simulink model "SemiActive_TS9"  (Simulink 7.6)
settings: Solver=ode45  SolverMode=SingleTasking  StartTime=0  StopTime=20  FixedStep=0.001  RelTol=1e-3  AbsTol=1e-6
libraries: Solver_SF x1
settings Model: Creator=bduprey  LastModifiedBy=mkhan  ExtModeTrigMode=oneshot  ExtModeArmWhenConnect=off
settings DataIOCC: LimitDataPoints=off  SignalLoggingName=sigsOut
settings OptimizationCC: BooleanDataType=off
settings DebuggingCC: SaveWithParameterizedLinksMsg=none  SignalResolutionControl=TryResolveAllWithWarning  SolverPrmCheckMsg=none  MultiTaskDSMMsg=warning  MultiTaskCondExecSysMsg=none  StrictBusMsg=None
settings HardwareCC: TargetUnknown=on
settings RTWCC: TemplateMakefile=grt_vc.tmf  IncludeERTFirstTime=on

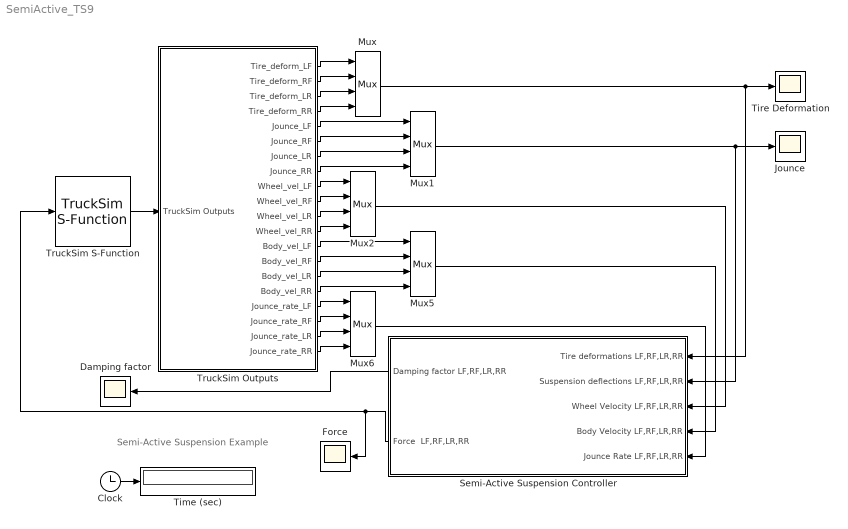
== system SemiActive_TS9 ==
  note: Semi-Active Suspension Example
  Clock : Clock
      settings: Decimation=10
  Damping factor : Scope
      settings: TickLabels=on  YMin=0  YMax=80000  DataFormat=Array  SampleTime=100
  Force : Scope
      settings: TickLabels=on  YMin=-100000  YMax=100000  DataFormat=Array  SampleTime=100
  Jounce : Scope
      settings: TickLabels=on  YMin=-0.1  YMax=0.3  DataFormat=Array  SampleTime=100
  Mux{,1..2,5..6} (5 alike) : Mux
  Semi-Active Suspension Controller : Subsystem  mask{K1=884.4, K1_R=679.6, K2=8624.1, K2_R=8624.1, K3=1398.9, K3_R=1924.8, K4=-5975.4, K4_R=-7823.4, SP_F=250000, SP_R=700000, OFF_F=0, OFF_R=0, GAIN1=0.8, GAIN2=2, UPLIM=400000, LWLIM=50}
      mask prompts: K1 "Optimal control gain, K1 (front)"; K1_R "Optimal control gain, K1 (rear)"; K2 "Optimal control gain, K2 (front)"; K2_R "Optimal control gain, K2 (rear)"; K3 "Optimal control gain, K3 (front)"; K3_R "Optimal control gain, K3 (rear)"; K4 "Optimal control gain, K4 (front)"; K4_R "Optimal control gain, K4 (rear)"; SP_F "Spring stiffness (front)  (N/m)"; SP_R "Spring stiffness (rear)  (N/m)"; OFF_F "Spring offset load (front) (N)"; OFF_R "Spring offset load (rear) (N)"; GAIN1 "Gain 1"; GAIN2 "Gain 2"; UPLIM "Variable damper upper limit (N-s/m)"; LWLIM "Variable damper lower limit (N-s/m)"
  Time (sec) : Display
      settings: Format=bank  Decimation=100
  Tire Deformation : Scope
      settings: TickLabels=on  YMin=-0.2  YMax=0.15  DataFormat=Array  SampleTime=100
  TruckSim Outputs : Subsystem
  TruckSim S-Function : Solver_SF/TruckSim S-Function  Priority=1  SIMFILE=simfile.sim
  wires:
  Mux2/1 -> Semi-Active Suspension Controller/3(Wheel Velocity LF,RF,LR,RR)
  Mux5/1 -> Semi-Active Suspension Controller/4(Body Velocity LF,RF,LR,RR)
  Mux/1 -> Semi-Active Suspension Controller/1(Tire deformations LF,RF,LR,RR), Tire Deformation/1
  Mux1/1 -> Semi-Active Suspension Controller/2(Suspension deflections LF,RF,LR,RR), Jounce/1
  Semi-Active Suspension Controller/1(Damping factor LF,RF,LR,RR) -> Damping factor/1
  Semi-Active Suspension Controller/2(Force  LF,RF,LR,RR) -> Force/1, TruckSim S-Function/1
  Mux6/1 -> Semi-Active Suspension Controller/5(Jounce Rate LF,RF,LR,RR)
  TruckSim S-Function/1 -> TruckSim Outputs/1(TruckSim Outputs)
  Clock/1 -> Time (sec)/1
  TruckSim Outputs/17(Jounce_rate_LF) -> Mux6/1
  TruckSim Outputs/18(Jounce_rate_RF) -> Mux6/2
  TruckSim Outputs/19(Jounce_rate_LR) -> Mux6/3
  TruckSim Outputs/20(Jounce_rate_RR) -> Mux6/4
  TruckSim Outputs/1(Tire_deform_LF) -> Mux/1
  TruckSim Outputs/2(Tire_deform_RF) -> Mux/2
  TruckSim Outputs/3(Tire_deform_LR) -> Mux/3
  TruckSim Outputs/4(Tire_deform_RR) -> Mux/4
  TruckSim Outputs/5(Jounce_LF) -> Mux1/1
  TruckSim Outputs/6(Jounce_RF) -> Mux1/2
  TruckSim Outputs/7(Jounce_LR) -> Mux1/3
  TruckSim Outputs/8(Jounce_RR) -> Mux1/4
  TruckSim Outputs/9(Wheel_vel_LF) -> Mux2/1
  TruckSim Outputs/10(Wheel_vel_RF) -> Mux2/2
  TruckSim Outputs/11(Wheel_vel_LR) -> Mux2/3
  TruckSim Outputs/12(Wheel_vel_RR) -> Mux2/4
  TruckSim Outputs/13(Body_vel_LF) -> Mux5/1
  TruckSim Outputs/14(Body_vel_RF) -> Mux5/2
  TruckSim Outputs/15(Body_vel_LR) -> Mux5/3
  TruckSim Outputs/16(Body_vel_RR) -> Mux5/4

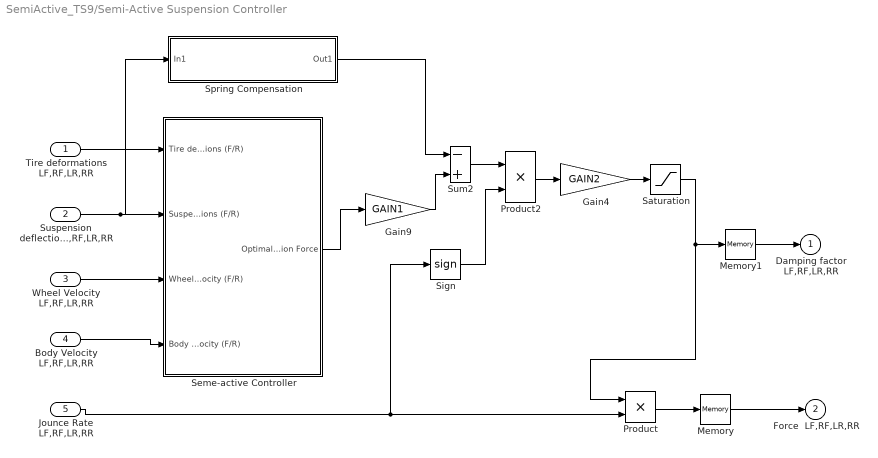
== system SemiActive_TS9/Semi-Active Suspension Controller ==
  Tire deformations LF,RF,LR,RR : Inport
  Suspension deflections LF,RF,LR,RR : Inport  Port=2
  Wheel Velocity LF,RF,LR,RR : Inport  Port=3
  Body Velocity LF,RF,LR,RR : Inport  Port=4
  Jounce Rate LF,RF,LR,RR : Inport  Port=5
  Gain4 : Gain  Gain=GAIN2  SaturateOnIntegerOverflow=on  OutDataTypeStr=Inherit: Same as input  ParamDataTypeStr=Inherit: Same as input
  Gain9 : Gain  Gain=GAIN1  SaturateOnIntegerOverflow=on  OutDataTypeStr=Inherit: Same as input  ParamDataTypeStr=Inherit: Same as input
  Memory : Memory
  Memory1 : Memory
  Product : Product  SaturateOnIntegerOverflow=on  InputSameDT=on  OutDataTypeStr=Inherit: Same as first input
  Product2 : Product  Inputs=**  SaturateOnIntegerOverflow=on  InputSameDT=on  OutDataTypeStr=Inherit: Same as first input
  Saturation : Saturate  UpperLimit=UPLIM  LowerLimit=LWLIM
  Seme-active Controller : Subsystem
  Sign : Signum
  Spring Compensation : Subsystem
  Sum2 : Sum  Inputs=-+  SaturateOnIntegerOverflow=on  InputSameDT=on  OutDataTypeStr=Inherit: Same as first input
  Damping factor LF,RF,LR,RR : Outport  InitialOutput=0
  Force  LF,RF,LR,RR : Outport  Port=2  InitialOutput=0
  wires:
  Tire deformations LF,RF,LR,RR/1 -> Seme-active Controller/1(Tire deformations (F/R))
  Body Velocity LF,RF,LR,RR/1 -> Seme-active Controller/4(Body Velocity (F/R))
  Wheel Velocity LF,RF,LR,RR/1 -> Seme-active Controller/3(Wheel Velocity (F/R))
  Jounce Rate LF,RF,LR,RR/1 -> Product/2, Sign/1
  Product/1 -> Memory/1
  Memory/1 -> Force  LF,RF,LR,RR/1
  Memory1/1 -> Damping factor LF,RF,LR,RR/1
  Suspension deflections LF,RF,LR,RR/1 -> Spring Compensation/1(In1), Seme-active Controller/2(Suspension deflections (F/R))
  Spring Compensation/1(Out1) -> Sum2/1
  Seme-active Controller/1(Optimal Suspension Force) -> Gain9/1
  Gain9/1 -> Sum2/2
  Product2/1 -> Gain4/1
  Sum2/1 -> Product2/1
  Sign/1 -> Product2/2
  Gain4/1 -> Saturation/1
  Saturation/1 -> Memory1/1, Product/1

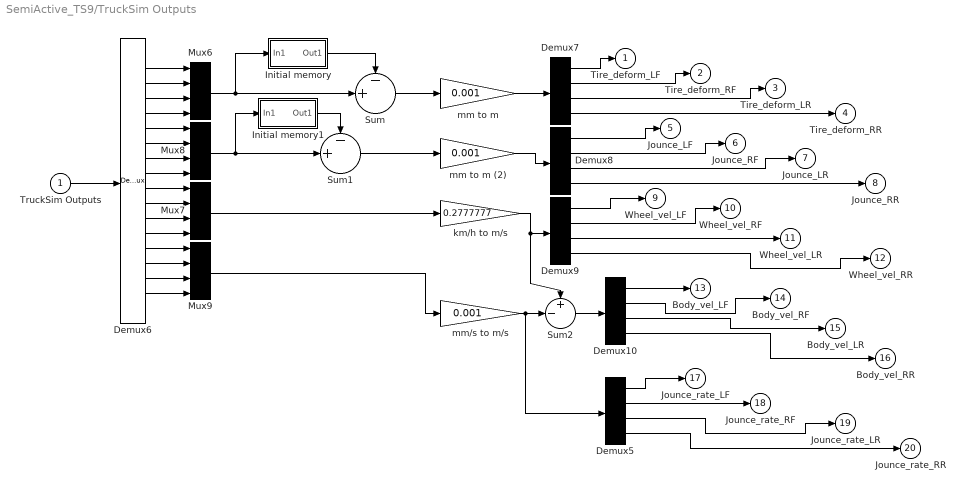
== system SemiActive_TS9/TruckSim Outputs ==
  TruckSim Outputs : Inport
  Demux{5,7..10} (5 alike) : Demux
  Demux6 : Demux  Outputs=16
  Initial memory : Subsystem
  Initial memory1 : Subsystem
  Mux{6..9} (4 alike) : Mux
  Sum : Sum  Inputs=-+|  SaturateOnIntegerOverflow=on
  Sum1 : Sum  Inputs=-+|  SaturateOnIntegerOverflow=on
  Sum2 : Sum  Inputs=+-|  SaturateOnIntegerOverflow=on  InputSameDT=on  OutDataTypeStr=Inherit: Same as first input
  km/h to m/s : Gain  Gain=0.2777777  SaturateOnIntegerOverflow=on  OutDataTypeStr=Inherit: Same as input  ParamDataTypeStr=Inherit: Same as input
  mm to m : Gain  Gain=0.001  SaturateOnIntegerOverflow=on  OutDataTypeStr=Inherit: Same as input  ParamDataTypeStr=Inherit: Same as input
  mm to m (2) : Gain  Gain=0.001  SaturateOnIntegerOverflow=on  OutDataTypeStr=Inherit: Same as input  ParamDataTypeStr=Inherit: Same as input
  mm/s to m/s : Gain  Gain=0.001  SaturateOnIntegerOverflow=on  OutDataTypeStr=Inherit: Same as input  ParamDataTypeStr=Inherit: Same as input
  Tire_deform_LF : Outport  InitialOutput=0
  Tire_deform_RF : Outport  Port=2  InitialOutput=0
  Tire_deform_LR : Outport  Port=3  InitialOutput=0
  Tire_deform_RR : Outport  Port=4  InitialOutput=0
  Jounce_LF : Outport  Port=5  InitialOutput=0
  Jounce_RF : Outport  Port=6  InitialOutput=0
  Jounce_LR : Outport  Port=7  InitialOutput=0
  Jounce_RR : Outport  Port=8  InitialOutput=0
  Wheel_vel_LF : Outport  Port=9  InitialOutput=0
  Wheel_vel_RF : Outport  Port=10  InitialOutput=0
  Wheel_vel_LR : Outport  Port=11  InitialOutput=0
  Wheel_vel_RR : Outport  Port=12  InitialOutput=0
  Body_vel_LF : Outport  Port=13  InitialOutput=0
  Body_vel_RF : Outport  Port=14  InitialOutput=0
  Body_vel_LR : Outport  Port=15  InitialOutput=0
  Body_vel_RR : Outport  Port=16  InitialOutput=0
  Jounce_rate_LF : Outport  Port=17  InitialOutput=0
  Jounce_rate_RF : Outport  Port=18  InitialOutput=0
  Jounce_rate_LR : Outport  Port=19  InitialOutput=0
  Jounce_rate_RR : Outport  Port=20  InitialOutput=0
  wires:
  Demux5/1 -> Jounce_rate_LF/1
  Demux5/2 -> Jounce_rate_RF/1
  Mux6/1 -> Initial memory/1(In1), Sum/2
  Demux7/1 -> Tire_deform_LF/1
  Demux7/2 -> Tire_deform_RF/1
  Demux7/3 -> Tire_deform_LR/1
  Demux7/4 -> Tire_deform_RR/1
  mm to m/1 -> Demux7/1
  Demux6/1 -> Mux6/1
  Demux6/2 -> Mux6/2
  Demux6/3 -> Mux6/3
  Demux6/4 -> Mux6/4
  mm to m (2)/1 -> Demux8/1
  Demux8/1 -> Jounce_LF/1
  Demux8/2 -> Jounce_RF/1
  Demux8/3 -> Jounce_LR/1
  Demux8/4 -> Jounce_RR/1
  Demux6/8 -> Mux8/4
  Demux6/7 -> Mux8/3
  Demux6/6 -> Mux8/2
  Demux6/5 -> Mux8/1
  Demux6/9 -> Mux7/1
  Demux6/10 -> Mux7/2
  Demux6/11 -> Mux7/3
  Demux6/12 -> Mux7/4
  Mux7/1 -> km/h to m/s/1
  km/h to m/s/1 -> Demux9/1, Sum2/1
  Demux9/1 -> Wheel_vel_LF/1
  Demux9/2 -> Wheel_vel_RF/1
  Demux9/3 -> Wheel_vel_LR/1
  Demux9/4 -> Wheel_vel_RR/1
  Demux6/13 -> Mux9/1
  Demux6/14 -> Mux9/2
  Demux6/15 -> Mux9/3
  Demux6/16 -> Mux9/4
  Mux9/1 -> mm/s to m/s/1
  mm/s to m/s/1 -> Sum2/2, Demux5/1
  Sum2/1 -> Demux10/1
  Demux10/1 -> Body_vel_LF/1
  Demux10/2 -> Body_vel_RF/1
  Demux10/3 -> Body_vel_LR/1
  Demux10/4 -> Body_vel_RR/1
  TruckSim Outputs/1 -> Demux6/1
  Demux5/3 -> Jounce_rate_LR/1
  Demux5/4 -> Jounce_rate_RR/1
  Initial memory/1(Out1) -> Sum/1
  Sum/1 -> mm to m/1
  Sum1/1 -> mm to m (2)/1
  Initial memory1/1(Out1) -> Sum1/1
  Mux8/1 -> Sum1/2, Initial memory1/1(In1)

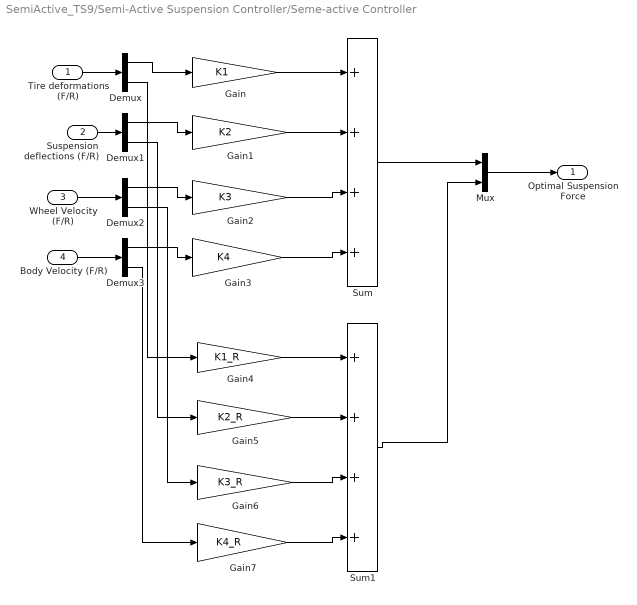
== system SemiActive_TS9/Semi-Active Suspension Controller/Seme-active Controller ==
  Tire deformations (F/R) : Inport
  Suspension deflections (F/R) : Inport  Port=2
  Wheel Velocity (F/R) : Inport  Port=3
  Body Velocity (F/R) : Inport  Port=4
  Demux{,1..3} (4 alike) : Demux  Outputs=[2 2]
  Gain : Gain  Gain=K1  SaturateOnIntegerOverflow=on  OutDataTypeStr=Inherit: Same as input  ParamDataTypeStr=Inherit: Same as input
  Gain1 : Gain  Gain=K2  SaturateOnIntegerOverflow=on  OutDataTypeStr=Inherit: Same as input  ParamDataTypeStr=Inherit: Same as input
  Gain2 : Gain  Gain=K3  SaturateOnIntegerOverflow=on  OutDataTypeStr=Inherit: Same as input  ParamDataTypeStr=Inherit: Same as input
  Gain3 : Gain  Gain=K4  SaturateOnIntegerOverflow=on  OutDataTypeStr=Inherit: Same as input  ParamDataTypeStr=Inherit: Same as input
  Gain4 : Gain  Gain=K1_R  SaturateOnIntegerOverflow=on  OutDataTypeStr=Inherit: Same as input  ParamDataTypeStr=Inherit: Same as input
  Gain5 : Gain  Gain=K2_R  SaturateOnIntegerOverflow=on  OutDataTypeStr=Inherit: Same as input  ParamDataTypeStr=Inherit: Same as input
  Gain6 : Gain  Gain=K3_R  SaturateOnIntegerOverflow=on  OutDataTypeStr=Inherit: Same as input  ParamDataTypeStr=Inherit: Same as input
  Gain7 : Gain  Gain=K4_R  SaturateOnIntegerOverflow=on  OutDataTypeStr=Inherit: Same as input  ParamDataTypeStr=Inherit: Same as input
  Mux : Mux  Inputs=2
  Sum : Sum  Inputs=++++  SaturateOnIntegerOverflow=on  InputSameDT=on  OutDataTypeStr=Inherit: Same as first input
  Sum1 : Sum  Inputs=++++  SaturateOnIntegerOverflow=on  InputSameDT=on  OutDataTypeStr=Inherit: Same as first input
  Optimal Suspension Force : Outport
  wires:
  Gain/1 -> Sum/1
  Gain1/1 -> Sum/2
  Gain2/1 -> Sum/3
  Gain3/1 -> Sum/4
  Tire deformations (F/R)/1 -> Demux/1
  Suspension deflections (F/R)/1 -> Demux1/1
  Wheel Velocity (F/R)/1 -> Demux2/1
  Body Velocity (F/R)/1 -> Demux3/1
  Gain4/1 -> Sum1/1
  Gain5/1 -> Sum1/2
  Gain6/1 -> Sum1/3
  Gain7/1 -> Sum1/4
  Sum1/1 -> Mux/2
  Demux/1 -> Gain/1
  Demux/2 -> Gain4/1
  Demux1/1 -> Gain1/1
  Demux1/2 -> Gain5/1
  Demux2/1 -> Gain2/1
  Demux2/2 -> Gain6/1
  Demux3/1 -> Gain3/1
  Demux3/2 -> Gain7/1
  Mux/1 -> Optimal Suspension Force/1
  Sum/1 -> Mux/1

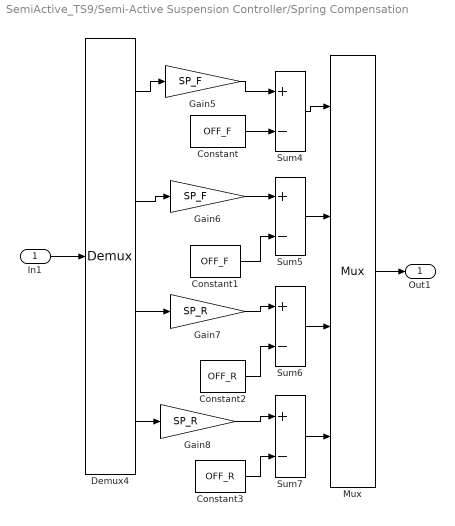
== system SemiActive_TS9/Semi-Active Suspension Controller/Spring Compensation ==
  In1 : Inport
  Constant : Constant  Value=OFF_F
  Constant1 : Constant  Value=OFF_F
  Constant2 : Constant  Value=OFF_R
  Constant3 : Constant  Value=OFF_R
  Demux4 : Demux
  Gain5 : Gain  Gain=SP_F  SaturateOnIntegerOverflow=on  OutDataTypeStr=Inherit: Same as input  ParamDataTypeStr=Inherit: Same as input
  Gain6 : Gain  Gain=SP_F  SaturateOnIntegerOverflow=on  OutDataTypeStr=Inherit: Same as input  ParamDataTypeStr=Inherit: Same as input
  Gain7 : Gain  Gain=SP_R  SaturateOnIntegerOverflow=on  OutDataTypeStr=Inherit: Same as input  ParamDataTypeStr=Inherit: Same as input
  Gain8 : Gain  Gain=SP_R  SaturateOnIntegerOverflow=on  OutDataTypeStr=Inherit: Same as input  ParamDataTypeStr=Inherit: Same as input
  Mux : Mux
  Sum{4..7} (4 alike) : Sum  Inputs=+-  SaturateOnIntegerOverflow=on  InputSameDT=on  OutDataTypeStr=Inherit: Same as first input
  Out1 : Outport
  wires:
  Demux4/1 -> Gain5/1
  Constant/1 -> Sum4/2
  Gain5/1 -> Sum4/1
  Constant1/1 -> Sum5/2
  Gain6/1 -> Sum5/1
  Demux4/2 -> Gain6/1
  Constant2/1 -> Sum6/2
  Gain7/1 -> Sum6/1
  Demux4/3 -> Gain7/1
  Demux4/4 -> Gain8/1
  Gain8/1 -> Sum7/1
  Constant3/1 -> Sum7/2
  Sum4/1 -> Mux/1
  Sum5/1 -> Mux/2
  Sum6/1 -> Mux/3
  Sum7/1 -> Mux/4
  In1/1 -> Demux4/1
  Mux/1 -> Out1/1

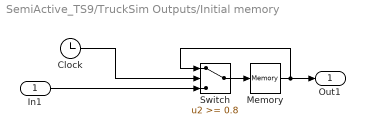
== system SemiActive_TS9/TruckSim Outputs/Initial memory ==
  In1 : Inport
  Clock : Clock
      settings: Decimation=10
  Memory : Memory
  Switch : Switch  Threshold=0.8  SaturateOnIntegerOverflow=on
  Out1 : Outport
  wires:
  Clock/1 -> Switch/2
  Memory/1 -> Out1/1, Switch/1
  Switch/1 -> Memory/1
  In1/1 -> Switch/3

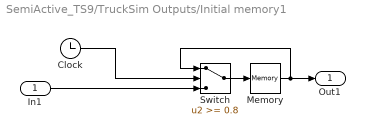
== system SemiActive_TS9/TruckSim Outputs/Initial memory1 ==
  In1 : Inport
  Clock : Clock
      settings: Decimation=10
  Memory : Memory
  Switch : Switch  Threshold=0.8  SaturateOnIntegerOverflow=on
  Out1 : Outport
  wires:
  Clock/1 -> Switch/2
  Memory/1 -> Out1/1, Switch/1
  Switch/1 -> Memory/1
  In1/1 -> Switch/3
